simulink model "mvardims_nonvirtualBus_fcnCallSS"  (Simulink 7.7)
settings: Solver=FixedStepDiscrete  StartTime=0.0  StopTime=10.0  FixedStep=0.2  RelTol=1e-3
PreLoadFcn:
  | load mvardims_bus2.mat;
libraries: simulink x1
CloseFcn:
  | clear a;
settings Model: Creator=djia  LastModifiedBy=kanantha  ExtModeAutoUpdateStatusClock=off
settings DataIOCC: SaveFormat=StructureWithTime
settings OptimizationCC: InlineParams=on  InitFltsAndDblsToZero=on  EfficientMapNaN2IntZero=off
settings DebuggingCC: UnderspecifiedInitializationDetection=Simplified
settings GRTTargetCC: TargetFcnLib=ansi_tfl_tmw.mat

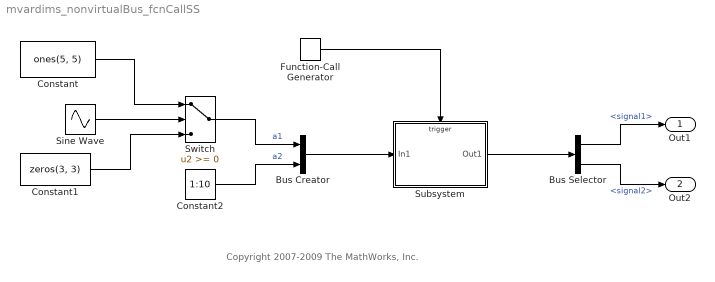
== system mvardims_nonvirtualBus_fcnCallSS ==
  note: Copyright 2007-2009 The MathWorks, Inc.
  Bus Creator : BusCreator  Inputs=2  OutDataTypeStr=Bus: a  NonVirtualBus=on
  Bus Selector : BusSelector  OutputSignals=signal1,signal2
  Constant : Constant  Value=ones(5, 5)
  Constant1 : Constant  Value=zeros(3, 3)
  Constant2 : Constant  Value=1:10  SampleTime=0.2
  Function-Call Generator : simulink/Ports & Subsystems/Function-Call Generator  sample_time=0.2  numberOfIterations=1
  Sine Wave : Sin  SampleTime=0.2
  Subsystem : Subsystem
  Switch : Switch  AllowDiffInputSizes=on
  Out1 : Outport
  Out2 : Outport  Port=2
  wires:
  Switch/1 -> Bus Creator/1  "a1"
  Constant/1 -> Switch/1
  Constant2/1 -> Bus Creator/2  "a2"
  Bus Selector/1 -> Out1/1  "<signal1>"
  Bus Selector/2 -> Out2/1  "<signal2>"
  Sine Wave/1 -> Switch/2
  Constant1/1 -> Switch/3
  Bus Creator/1 -> Subsystem/1(In1)
  Subsystem/1(Out1) -> Bus Selector/1
  Function-Call Generator/1 -> Subsystem/Trigger

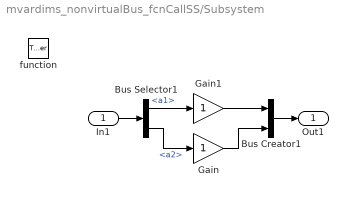
== system mvardims_nonvirtualBus_fcnCallSS/Subsystem ==
  In1 : Inport
  function : TriggerPort  TriggerType=function-call
  Bus Creator1 : BusCreator  Inputs=2  NonVirtualBus=on
  Bus Selector1 : BusSelector  OutputSignals=a1,a2
  Gain : Gain
  Gain1 : Gain
  Out1 : Outport  InitialOutput=0
  wires:
  Bus Selector1/1 -> Gain1/1  "<a1>"
  Bus Selector1/2 -> Gain/1  "<a2>"
  Gain/1 -> Bus Creator1/2
  Bus Creator1/1 -> Out1/1
  In1/1 -> Bus Selector1/1
  Gain1/1 -> Bus Creator1/1
